simulink model "attitude_delay_mdl"  (Simulink 7.0)
settings: Solver=ode4  SolverMode=SingleTasking  StartTime=0.0  StopTime=tdur  FixedStep=dt  RelTol=1e-3
values from neighbouring files (symbols this model uses):
  dt = 0.1    [attitude_controller_response.m]
  I = I_array(ax)    [attitude_controller_response.m]
  Kd = Kd_array(ax)    [attitude_controller_response.m]
  Kp = Kp_array(ax)    [attitude_controller_response.m]
  Krcs = 1    [attitude_controller_response.m]
  t_delay = 10    [attitude_controller_response.m]
  Tdist = Tdist_array(ax)    [attitude_controller_response.m]
  Trcs_max = Trcs_max_array(ax)    [attitude_controller_response.m]
libraries: simulink_extras x2
settings Model: Creator=hardac_s  LastModifiedBy=hardac_s
settings DataIOCC: LimitDataPoints=off  SaveOutput=off  SignalLoggingName=sigsOut
settings DebuggingCC: SaveWithParameterizedLinksMsg=none  SignalResolutionControl=TryResolveAllWithWarning  SolverPrmCheckMsg=none  MultiTaskDSMMsg=warning  MultiTaskCondExecSysMsg=none  StrictBusMsg=None
settings HardwareCC: TargetUnknown=on
settings RTWCC: IncludeERTFirstTime=on

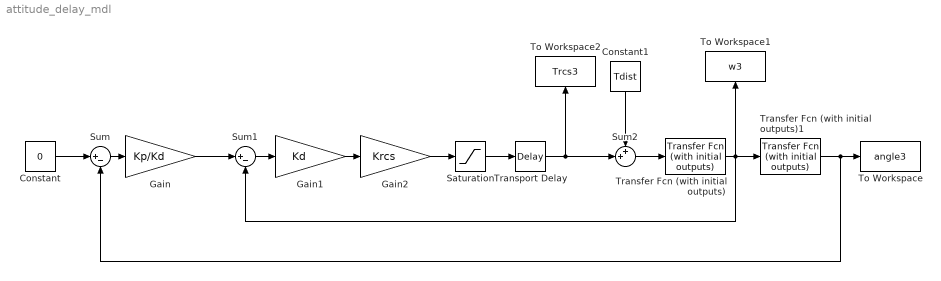
== system attitude_delay_mdl ==
  Constant : Constant  Value=0  OutDataType=sfix(16)  OutScaling=2^0
  Constant1 : Constant  Orientation=down  Value=Tdist  OutDataType=sfix(16)  OutScaling=2^0
  Gain : Gain  Gain=Kp/Kd  ParameterDataType=sfix(16)  ParameterScaling=2^0  OutDataType=sfix(16)  OutScaling=2^0  SaturateOnIntegerOverflow=on
  Gain1 : Gain  Gain=Kd  ParameterDataType=sfix(16)  ParameterScaling=2^0  OutDataType=sfix(16)  OutScaling=2^0  SaturateOnIntegerOverflow=on
  Gain2 : Gain  Gain=Krcs  ParameterDataType=sfix(16)  ParameterScaling=2^0  OutDataType=sfix(16)  OutScaling=2^0  SaturateOnIntegerOverflow=on
  Saturation : Saturate  UpperLimit=Trcs_max  LowerLimit=-Trcs_max  SampleTime=dt
  Sum : Sum  Inputs=|+-  OutDataType=sfix(16)  OutScaling=2^0  SaturateOnIntegerOverflow=on
  Sum1 : Sum  Inputs=|+-  OutDataType=sfix(16)  OutScaling=2^0  SaturateOnIntegerOverflow=on
  Sum2 : Sum  Inputs=++|  OutDataType=sfix(16)  OutScaling=2^0  SaturateOnIntegerOverflow=on
  To Workspace : ToWorkspace  VariableName=angle3  SampleTime=dt  SaveFormat=Array
  To Workspace1 : ToWorkspace  VariableName=w3  SampleTime=dt  SaveFormat=Array
      settings: Orientation=up
  To Workspace2 : ToWorkspace  VariableName=Trcs3  SampleTime=dt  SaveFormat=Array
      settings: Orientation=up
  Transfer Fcn (with initial outputs) : simulink_extras/Additional Linear/Transfer Fcn (with initial outputs)  SystemSampleTime=-1  N=[1]  D=[I 0]  Y0=w0  U0=0
  Transfer Fcn (with initial outputs)1 : simulink_extras/Additional Linear/Transfer Fcn (with initial outputs)  SystemSampleTime=-1  N=[1]  D=[1 0]  Y0=angle0  U0=w0
  Transport Delay : TransportDelay  DelayTime=t_delay
  wires:
  Sum/1 -> Gain/1
  Constant/1 -> Sum/1
  Gain/1 -> Sum1/1
  Sum1/1 -> Gain1/1
  Gain1/1 -> Gain2/1
  Transfer Fcn (with initial outputs)/1 -> Transfer Fcn (with initial outputs)1/1, Sum1/2, To Workspace1/1
  Transfer Fcn (with initial outputs)1/1 -> Sum/2, To Workspace/1
  Sum2/1 -> Transfer Fcn (with initial outputs)/1
  Gain2/1 -> Saturation/1
  Constant1/1 -> Sum2/1
  Transport Delay/1 -> Sum2/2, To Workspace2/1
  Saturation/1 -> Transport Delay/1
